simulink model "UKF_nav"  (R2018b)
settings: Solver=ode4  StartTime=0.0  StopTime=SimEndTime  FixedStep=TimeStep  RelTol=1e-3
model workspace (MATLAB code in the model file):
  | CON = Simulink.Parameter;
  | CON.DataType = 'Bus: Bus_CON';
  | CON.Value = Simulink.Bus.createMATLABStruct('Bus_CON');
undefined symbols (not defined in the file): computer_dt, SampleTime
libraries: simulink x1
settings Model: ParameterArgumentNames=CON  OrderedModelArguments=off  Creator=Ethan  LastModifiedBy=Ethan
settings ModelReferenceCC: ModelReferenceNumInstancesAllowed=Single

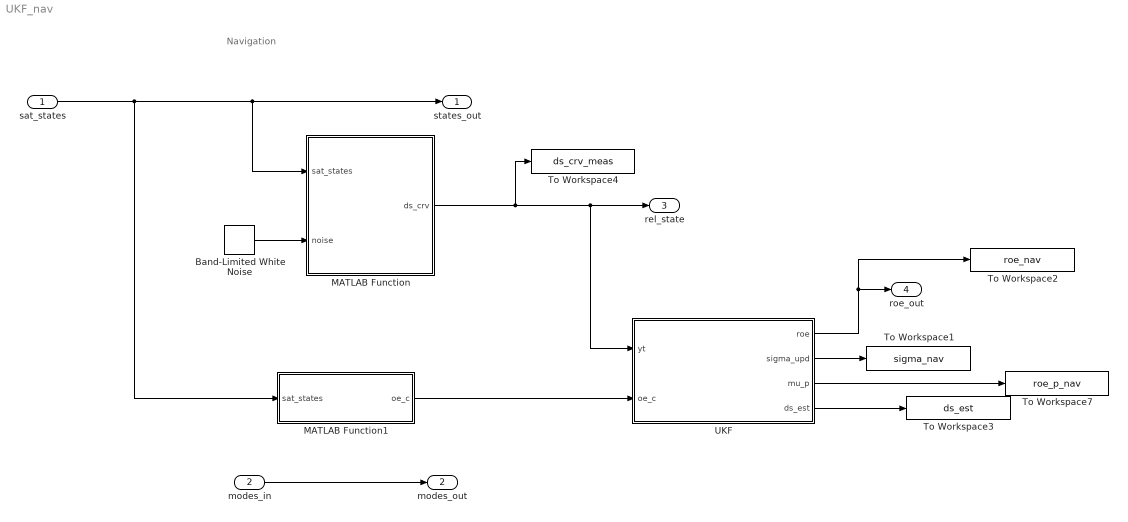
== system UKF_nav ==
  note: Navigation
  sat_states : Inport  OutDataTypeStr=Bus: Bus_outputs
  modes_in : Inport  Port=2  OutDataTypeStr=Bus: Bus_modes
  Band-Limited White Noise : simulink/Sources/Band-Limited White Noise  Cov=[0.000001; 0.000001; 0.000001; 0.000000001; 0.000000001; 0.000000001]/1000  Ts=computer_dt  seed=[23341, 23342, 23343, 23344, 23345, 23346]
  MATLAB Function : MATLAB Function  TreatAsAtomicUnit=on
  MATLAB Function1 : MATLAB Function  TreatAsAtomicUnit=on
  To Workspace1 : ToWorkspace  VariableName=sigma_nav  SaveFormat=Timeseries  SampleTime=SampleTime
      settings: Save2DSignal=2-D array (concatenate along first dimension)
  To Workspace2 : ToWorkspace  VariableName=roe_nav  SaveFormat=Timeseries  SampleTime=SampleTime
      settings: Save2DSignal=2-D array (concatenate along first dimension)
  To Workspace3 : ToWorkspace  VariableName=ds_est  SampleTime=SampleTime
      settings: Save2DSignal=2-D array (concatenate along first dimension)
  To Workspace4 : ToWorkspace  VariableName=ds_crv_meas  SaveFormat=Timeseries  SampleTime=SampleTime
      settings: Save2DSignal=2-D array (concatenate along first dimension)
  To Workspace7 : ToWorkspace  VariableName=roe_p_nav  SaveFormat=Timeseries  SampleTime=SampleTime
      settings: Save2DSignal=2-D array (concatenate along first dimension)
  UKF : MATLAB Function  TreatAsAtomicUnit=on
  states_out : Outport  OutDataTypeStr=Bus: Bus_outputs
  modes_out : Outport  Port=2  OutDataTypeStr=Bus: Bus_modes
  rel_state : Outport  Port=3
  roe_out : Outport  Port=4  OutDataTypeStr=Bus: Bus_roe
  wires:
  modes_in/1 -> modes_out/1
  sat_states/1 -> MATLAB Function1/1(sat_states), MATLAB Function/1(sat_states), states_out/1
  UKF/1(roe) -> To Workspace2/1, roe_out/1
  UKF/3(mu_p) -> To Workspace7/1
  UKF/2(sigma_upd) -> To Workspace1/1
  MATLAB Function1/1(oe_c) -> UKF/2(oe_c)
  MATLAB Function/1(ds_crv) -> To Workspace4/1, UKF/1(yt), rel_state/1
  Band-Limited White Noise/1 -> MATLAB Function/2(noise)
  UKF/4(ds_est) -> To Workspace3/1

== matlab function UKF_nav/MATLAB Function1 ==
  data: sat_states input; oe_c output Bus: Bus_OE; CON parameter
function oe_c = fcn(sat_states, CON)
deg2rad = pi / 180;
chief = sat_states.NXS_out;
[oe_c.a, oe_c.e, oe_c.inc, oe_c.omega, oe_c.w, oe_c.nu, ~] = ECI2OE(chief.r_i, chief.v_i, CON.mu);


% moe_c = osc2mean([oe_c.a, oe_c.e, oe_c.inc, oe_c.omega, oe_c.w, oe_c.nu], CON.Re, CON.J2);
oe_c.inc = oe_c.inc * deg2rad;
oe_c.omega = oe_c.omega * deg2rad;
oe_c.w = oe_c.w * deg2rad;
oe_c.nu = oe_c.nu * deg2rad;

% oe_c.a = moe_c(1);
% oe_c.e = moe_c(2);
% oe_c.inc = deg2rad * moe_c(3);
% oe_c.omega = deg2rad * moe_c(4);
% oe_c.w = deg2rad * moe_c(5);
% oe_c.nu = deg2rad * moe_c(6);



end

== matlab function UKF_nav/MATLAB Function ==
  data: sat_states input; ds_crv output; noise input
function ds_crv  = i2relRTN(sat_states, noise)

chief = sat_states.NXS_out;
deputy = sat_states.astro_out;

[rHill,vHill] = ECI2Hill_Vectorized(chief.r_i,chief.v_i,deputy.r_i,deputy.v_i);
ds_crv = [rHill;vHill];
% ds_crv = ds_crv + [0.001; 0.001; 0.00001; 0.00001; 0.00001;0.00001];
ds_crv = ds_crv + noise;
end

== matlab function UKF_nav/UKF ==
  data: yt input; roe output Bus: Bus_roe; oe_c input; sigma_upd output; mu_p output; CON parameter; ds_est output
function [roe, sigma_upd, mu_p, ds_est] = UKF(yt, oe_c, CON)

%%
% yt is the noisy measurement [rel_pos; rel_vel];

%% Initialization
persistent sigma_prev mu_prev Rt Qt
if isempty(mu_prev)
    
    mu_prev = ones(7, 1)  * 0.0001;
    mu_prev(1) = -4.5075e-10;
    mu_prev(3) = 0;
%     mu_prev = [0; 1e-4; 1e-6; 1e-7; 1e-8; 1e-10; 1e-12];
    Qt = CON.Qt;
    Rt = CON.Rt;
end


%% UKF, Predict
if isempty(sigma_prev)
   sigma_prev = eye(7) * 1e-3;
end


[x_p, w_p] = UT(mu_prev, sigma_prev, CON.lambda);
x_p_bar = zeros(size(x_p));
for ii = 1:size(x_p, 2)
    state = x_p(:, ii);
    A = roe_state_matrix_UKF(sqrt(CON.mu / oe_c.a^3), CON.computer_dt, oe_c, CON);
    x_p_bar(:, ii) = A * state;
end

[mu_p, sigma_bar] = UT_inv(x_p_bar, w_p);
sigma_p = sigma_bar + Qt;

%% UKF, Update
[x_p, w_p] = UT(mu_p, sigma_p, CON.lambda);
y_fake = zeros(size(x_p, 2), 6);
y_hat = zeros(6, 1);
for ii = 1 : size(x_p, 2)
    y_fake(ii, :) = roe2Hill(x_p(:, ii), oe_c);
    y_hat = y_hat + w_p(ii) * y_fake(ii, :)';
end


E_y = zeros(size(y_hat, 1), size(y_hat, 1));
E_xy = zeros(size(mu_p, 1), size(y_hat, 1));

for jj = 1:size(x_p, 2)
    E_y = E_y + w_p(jj)*(y_fake(jj, :)' - y_hat) * (y_fake(jj, :)' - y_hat)';
    E_xy = E_xy + w_p(jj) * (x_p(:, jj) - mu_p) * (y_fake(jj, :)' - y_hat)';
end
E_y = E_y + Rt;

mu_upd = mu_p + E_xy * E_y^(-1) * (yt - y_hat);
sigma_upd = sigma_p - E_xy * E_y^(-1) * E_xy';

mu_upd(1) = -4.5075e-10;
mu_prev = mu_upd;
sigma_prev = sigma_upd;

roe.adot = mu_upd(1);
roe.da = mu_upd(2);
roe.dL = mu_upd(3);
roe.dex = mu_upd(4);
roe.dey = mu_upd(5);
roe.dix = mu_upd(6);
roe.diy = mu_upd(7);
ds_est = roe2Hill(mu_upd, oe_c);
end
